simulink model "dds_cwg"  (R2016b)
settings: Solver=VariableStepAuto  StartTime=0.0  StopTime=2048*10  RelTol=1e-3
undefined symbols (not defined in the file or in its folder): fft_stages, n_taps
undefined symbols (not defined in the file): Coeffs, pfb_coeff_gen_calc
libraries: xbsIndex_r4 x6830, casper_library_misc x16, casper_library_delays x2
(part 15 of 67)

== system dds_cwg/DDC/dec_fir_async ==
  sync_in : Inport
  dv_in : Inport  Port=2
  real1 : Inport  Port=3
  imag1 : Inport  Port=4
  real2 : Inport  Port=5
  imag2 : Inport  Port=6
  real3 : Inport  Port=7
  imag3 : Inport  Port=8
  real4 : Inport  Port=9
  imag4 : Inport  Port=10
  real5 : Inport  Port=11
  imag5 : Inport  Port=12
  real6 : Inport  Port=13
  imag6 : Inport  Port=14
  real7 : Inport  Port=15
  imag7 : Inport  Port=16
  real8 : Inport  Port=17
  imag8 : Inport  Port=18
  convert1 : xbsIndex_r4/Convert  gui_display_data_type=Fixed-point  arith_type="Signed  (2's comp)"  n_bits=35  bin_pt=26  float_type=Single  exp_bits=8  fraction_bits=24  quantization="Round  (unbiased: +/- Inf)"  overflow=Wrap  en=off  latency=7  pipeline=off  dbl_ovrd=off  block_type=convert
  convert2 : xbsIndex_r4/Convert  gui_display_data_type=Fixed-point  arith_type="Signed  (2's comp)"  n_bits=35  bin_pt=26  float_type=Single  exp_bits=8  fraction_bits=24  quantization="Round  (unbiased: +/- Inf)"  overflow=Wrap  en=off  latency=7  pipeline=off  dbl_ovrd=off  block_type=convert
  dv_delay : xbsIndex_r4/Delay  rst=off  infoeditControl=Selection of Reset will increase slice count due to use of real FFs and instead of SRLs  en=off  latency=70  reg_retiming=off  dbl_ovrd=off  block_type=delay
      settings: infoedit=Hardware notes: A delay line is a chain, each link of which is an SRL16 or SRL32 followed by a flip-flop.
  fir_col_async1 : Subsystem  AncestorBlock=casper_library_downconverter/fir_col_async  mask(fir_col_async){n_inputs=8, coeff=[-0.0012628 -0.00099956 -0.00074444 -0.00051594 -0.00032729 -0.00018718 -0.00010242  0.00015765], add_latency=7, mult_latency=7, coeff_bit_width=18, coeff_bin_pt=17, first_stage_hdl=on, adder_imp=DSP48, async=on, bus_input=off, input_width=0, input_bp=0, input_type=Signed, dbl=off}
      mask prompts: n_inputs "Inputs"; coeff "Coefficients"; add_latency "Add latency"; mult_latency "Mult Latency"; coeff_bit_width "Coefficient bit width"; coeff_bin_pt "Coefficient binary point"; first_stage_hdl "Implement first stage of adder trees on output as behavioural HDL"; adder_imp "Adder implementation"; async "Asynchronous ops"; bus_input "Bus input"; input_width "Input bitwidth"; input_bp "Input binary point"; input_type "Input datatype"; dbl "Double col"
      mask init:
      | fir_col_async_init(gcb);
      mask Help: eval('xlWeb(''http://casper.berkeley.edu/wiki/Fir_col'')')
      mask TypeOptions adder_imp: Behavioral | Fabric | DSP48
      mask Callback bus_input:
      | onoff = get_param(gcb, 'bus_input');
      | set_param_state(gcb, 'input_width', onoff)
      | set_param_state(gcb, 'input_bp', onoff)
      | set_param_state(gcb, 'input_type', onoff)
      mask TypeOptions input_type: Signed | Unsigned
  fir_col_async10 : Subsystem  AncestorBlock=casper_library_downconverter/fir_col_async  mask(fir_col_async){n_inputs=8, coeff=[0.070166    0.055743    0.040656     0.02581    0.012049  9.3633e-05  -0.0095102   -0.016422], add_latency=7, mult_latency=7, coeff_bit_width=18, coeff_bin_pt=17, first_stage_hdl=on, adder_imp=DSP48, async=on, bus_input=off, input_width=0, input_bp=0, input_type=Signed, dbl=off}
      mask prompts: n_inputs "Inputs"; coeff "Coefficients"; add_latency "Add latency"; mult_latency "Mult Latency"; coeff_bit_width "Coefficient bit width"; coeff_bin_pt "Coefficient binary point"; first_stage_hdl "Implement first stage of adder trees on output as behavioural HDL"; adder_imp "Adder implementation"; async "Asynchronous ops"; bus_input "Bus input"; input_width "Input bitwidth"; input_bp "Input binary point"; input_type "Input datatype"; dbl "Double col"
      mask init:
      | fir_col_async_init(gcb);
      mask Help: eval('xlWeb(''http://casper.berkeley.edu/wiki/Fir_col'')')
      mask TypeOptions adder_imp: Behavioral | Fabric | DSP48
      mask Callback bus_input:
      | onoff = get_param(gcb, 'bus_input');
      | set_param_state(gcb, 'input_width', onoff)
      | set_param_state(gcb, 'input_bp', onoff)
      | set_param_state(gcb, 'input_type', onoff)
      mask TypeOptions input_type: Signed | Unsigned
  fir_col_async11 : Subsystem  AncestorBlock=casper_library_downconverter/fir_col_async  mask(fir_col_async){n_inputs=8, coeff=[0.083023    0.093488     0.10088      0.1047      0.1047     0.10088    0.093488    0.083023], add_latency=7, mult_latency=7, coeff_bit_width=18, coeff_bin_pt=17, first_stage_hdl=on, adder_imp=DSP48, async=on, bus_input=off, input_width=0, input_bp=0, input_type=Signed, dbl=off}
      mask prompts: n_inputs "Inputs"; coeff "Coefficients"; add_latency "Add latency"; mult_latency "Mult Latency"; coeff_bit_width "Coefficient bit width"; coeff_bin_pt "Coefficient binary point"; first_stage_hdl "Implement first stage of adder trees on output as behavioural HDL"; adder_imp "Adder implementation"; async "Asynchronous ops"; bus_input "Bus input"; input_width "Input bitwidth"; input_bp "Input binary point"; input_type "Input datatype"; dbl "Double col"
      mask init:
      | fir_col_async_init(gcb);
      mask Help: eval('xlWeb(''http://casper.berkeley.edu/wiki/Fir_col'')')
      mask TypeOptions adder_imp: Behavioral | Fabric | DSP48
      mask Callback bus_input:
      | onoff = get_param(gcb, 'bus_input');
      | set_param_state(gcb, 'input_width', onoff)
      | set_param_state(gcb, 'input_bp', onoff)
      | set_param_state(gcb, 'input_type', onoff)
      mask TypeOptions input_type: Signed | Unsigned
  fir_col_async12 : Subsystem  AncestorBlock=casper_library_downconverter/fir_col_async  mask(fir_col_async){n_inputs=8, coeff=[-0.016422  -0.0095102  9.3633e-05    0.012049     0.02581    0.040656    0.055743    0.070166], add_latency=7, mult_latency=7, coeff_bit_width=18, coeff_bin_pt=17, first_stage_hdl=on, adder_imp=DSP48, async=on, bus_input=off, input_width=0, input_bp=0, input_type=Signed, dbl=off}
      mask prompts: n_inputs "Inputs"; coeff "Coefficients"; add_latency "Add latency"; mult_latency "Mult Latency"; coeff_bit_width "Coefficient bit width"; coeff_bin_pt "Coefficient binary point"; first_stage_hdl "Implement first stage of adder trees on output as behavioural HDL"; adder_imp "Adder implementation"; async "Asynchronous ops"; bus_input "Bus input"; input_width "Input bitwidth"; input_bp "Input binary point"; input_type "Input datatype"; dbl "Double col"
      mask init:
      | fir_col_async_init(gcb);
      mask Help: eval('xlWeb(''http://casper.berkeley.edu/wiki/Fir_col'')')
      mask TypeOptions adder_imp: Behavioral | Fabric | DSP48
      mask Callback bus_input:
      | onoff = get_param(gcb, 'bus_input');
      | set_param_state(gcb, 'input_width', onoff)
      | set_param_state(gcb, 'input_bp', onoff)
      | set_param_state(gcb, 'input_type', onoff)
      mask TypeOptions input_type: Signed | Unsigned
  fir_col_async13 : Subsystem  AncestorBlock=casper_library_downconverter/fir_col_async  mask(fir_col_async){n_inputs=8, coeff=[0.0023352  -0.0027452  -0.0081837   -0.013424   -0.017857    -0.02087   -0.021908   -0.020523], add_latency=7, mult_latency=7, coeff_bit_width=18, coeff_bin_pt=17, first_stage_hdl=on, adder_imp=DSP48, async=on, bus_input=off, input_width=0, input_bp=0, input_type=Signed, dbl=off}
      mask prompts: n_inputs "Inputs"; coeff "Coefficients"; add_latency "Add latency"; mult_latency "Mult Latency"; coeff_bit_width "Coefficient bit width"; coeff_bin_pt "Coefficient binary point"; first_stage_hdl "Implement first stage of adder trees on output as behavioural HDL"; adder_imp "Adder implementation"; async "Asynchronous ops"; bus_input "Bus input"; input_width "Input bitwidth"; input_bp "Input binary point"; input_type "Input datatype"; dbl "Double col"
      mask init:
      | fir_col_async_init(gcb);
      mask Help: eval('xlWeb(''http://casper.berkeley.edu/wiki/Fir_col'')')
      mask TypeOptions adder_imp: Behavioral | Fabric | DSP48
      mask Callback bus_input:
      | onoff = get_param(gcb, 'bus_input');
      | set_param_state(gcb, 'input_width', onoff)
      | set_param_state(gcb, 'input_bp', onoff)
      | set_param_state(gcb, 'input_type', onoff)
      mask TypeOptions input_type: Signed | Unsigned
  fir_col_async14 : Subsystem  AncestorBlock=casper_library_downconverter/fir_col_async  mask(fir_col_async){n_inputs=8, coeff=[0.0033255   0.0064163   0.0090972    0.011022     0.01189    0.011487     0.00971   0.0065975], add_latency=7, mult_latency=7, coeff_bit_width=18, coeff_bin_pt=17, first_stage_hdl=on, adder_imp=DSP48, async=on, bus_input=off, input_width=0, input_bp=0, input_type=Signed, dbl=off}
      mask prompts: n_inputs "Inputs"; coeff "Coefficients"; add_latency "Add latency"; mult_latency "Mult Latency"; coeff_bit_width "Coefficient bit width"; coeff_bin_pt "Coefficient binary point"; first_stage_hdl "Implement first stage of adder trees on output as behavioural HDL"; adder_imp "Adder implementation"; async "Asynchronous ops"; bus_input "Bus input"; input_width "Input bitwidth"; input_bp "Input binary point"; input_type "Input datatype"; dbl "Double col"
      mask init:
      | fir_col_async_init(gcb);
      mask Help: eval('xlWeb(''http://casper.berkeley.edu/wiki/Fir_col'')')
      mask TypeOptions adder_imp: Behavioral | Fabric | DSP48
      mask Callback bus_input:
      | onoff = get_param(gcb, 'bus_input');
      | set_param_state(gcb, 'input_width', onoff)
      | set_param_state(gcb, 'input_bp', onoff)
      | set_param_state(gcb, 'input_type', onoff)
      mask TypeOptions input_type: Signed | Unsigned
  fir_col_async15 : Subsystem  AncestorBlock=casper_library_downconverter/fir_col_async  mask(fir_col_async){n_inputs=8, coeff=[-0.0050789  -0.0065053  -0.0073276  -0.0073948  -0.0066259  -0.0050262  -0.0026942  0.00017956], add_latency=7, mult_latency=7, coeff_bit_width=18, coeff_bin_pt=17, first_stage_hdl=on, adder_imp=DSP48, async=on, bus_input=off, input_width=0, input_bp=0, input_type=Signed, dbl=off}
      mask prompts: n_inputs "Inputs"; coeff "Coefficients"; add_latency "Add latency"; mult_latency "Mult Latency"; coeff_bit_width "Coefficient bit width"; coeff_bin_pt "Coefficient binary point"; first_stage_hdl "Implement first stage of adder trees on output as behavioural HDL"; adder_imp "Adder implementation"; async "Asynchronous ops"; bus_input "Bus input"; input_width "Input bitwidth"; input_bp "Input binary point"; input_type "Input datatype"; dbl "Double col"
      mask init:
      | fir_col_async_init(gcb);
      mask Help: eval('xlWeb(''http://casper.berkeley.edu/wiki/Fir_col'')')
      mask TypeOptions adder_imp: Behavioral | Fabric | DSP48
      mask Callback bus_input:
      | onoff = get_param(gcb, 'bus_input');
      | set_param_state(gcb, 'input_width', onoff)
      | set_param_state(gcb, 'input_bp', onoff)
      | set_param_state(gcb, 'input_type', onoff)
      mask TypeOptions input_type: Signed | Unsigned
  fir_col_async16 : Subsystem  AncestorBlock=casper_library_downconverter/fir_col_async  mask(fir_col_async){n_inputs=8, coeff=[0.0046187    0.004871   0.0045962   0.0037763   0.0024531  0.00072919  -0.0012378  -0.0032483], add_latency=7, mult_latency=7, coeff_bit_width=18, coeff_bin_pt=17, first_stage_hdl=on, adder_imp=DSP48, async=on, bus_input=off, input_width=0, input_bp=0, input_type=Signed, dbl=off}
      mask prompts: n_inputs "Inputs"; coeff "Coefficients"; add_latency "Add latency"; mult_latency "Mult Latency"; coeff_bit_width "Coefficient bit width"; coeff_bin_pt "Coefficient binary point"; first_stage_hdl "Implement first stage of adder trees on output as behavioural HDL"; adder_imp "Adder implementation"; async "Asynchronous ops"; bus_input "Bus input"; input_width "Input bitwidth"; input_bp "Input binary point"; input_type "Input datatype"; dbl "Double col"
      mask init:
      | fir_col_async_init(gcb);
      mask Help: eval('xlWeb(''http://casper.berkeley.edu/wiki/Fir_col'')')
      mask TypeOptions adder_imp: Behavioral | Fabric | DSP48
      mask Callback bus_input:
      | onoff = get_param(gcb, 'bus_input');
      | set_param_state(gcb, 'input_width', onoff)
      | set_param_state(gcb, 'input_bp', onoff)
      | set_param_state(gcb, 'input_type', onoff)
      mask TypeOptions input_type: Signed | Unsigned
  fir_col_async17 : Subsystem  AncestorBlock=casper_library_downconverter/fir_col_async  mask(fir_col_async){n_inputs=8, coeff=[-0.0031192  -0.0027219  -0.0019821 -0.00095069  0.00028337   0.0015999   0.0028581   0.0039104], add_latency=7, mult_latency=7, coeff_bit_width=18, coeff_bin_pt=17, first_stage_hdl=on, adder_imp=DSP48, async=on, bus_input=off, input_width=0, input_bp=0, input_type=Signed, dbl=off}
      mask prompts: n_inputs "Inputs"; coeff "Coefficients"; add_latency "Add latency"; mult_latency "Mult Latency"; coeff_bit_width "Coefficient bit width"; coeff_bin_pt "Coefficient binary point"; first_stage_hdl "Implement first stage of adder trees on output as behavioural HDL"; adder_imp "Adder implementation"; async "Asynchronous ops"; bus_input "Bus input"; input_width "Input bitwidth"; input_bp "Input binary point"; input_type "Input datatype"; dbl "Double col"
      mask init:
      | fir_col_async_init(gcb);
      mask Help: eval('xlWeb(''http://casper.berkeley.edu/wiki/Fir_col'')')
      mask TypeOptions adder_imp: Behavioral | Fabric | DSP48
      mask Callback bus_input:
      | onoff = get_param(gcb, 'bus_input');
      | set_param_state(gcb, 'input_width', onoff)
      | set_param_state(gcb, 'input_bp', onoff)
      | set_param_state(gcb, 'input_type', onoff)
      mask TypeOptions input_type: Signed | Unsigned
  fir_col_async18 : Subsystem  AncestorBlock=casper_library_downconverter/fir_col_async  mask(fir_col_async){n_inputs=8, coeff=[0.00149  0.00087891  0.00011449 -0.00073276  -0.0015765  -0.0023222  -0.0028776  -0.0031624], add_latency=7, mult_latency=7, coeff_bit_width=18, coeff_bin_pt=17, first_stage_hdl=on, adder_imp=DSP48, async=on, bus_input=off, input_width=0, input_bp=0, input_type=Signed, dbl=off}
      mask prompts: n_inputs "Inputs"; coeff "Coefficients"; add_latency "Add latency"; mult_latency "Mult Latency"; coeff_bit_width "Coefficient bit width"; coeff_bin_pt "Coefficient binary point"; first_stage_hdl "Implement first stage of adder trees on output as behavioural HDL"; adder_imp "Adder implementation"; async "Asynchronous ops"; bus_input "Bus input"; input_width "Input bitwidth"; input_bp "Input binary point"; input_type "Input datatype"; dbl "Double col"
      mask init:
      | fir_col_async_init(gcb);
      mask Help: eval('xlWeb(''http://casper.berkeley.edu/wiki/Fir_col'')')
      mask TypeOptions adder_imp: Behavioral | Fabric | DSP48
      mask Callback bus_input:
      | onoff = get_param(gcb, 'bus_input');
      | set_param_state(gcb, 'input_width', onoff)
      | set_param_state(gcb, 'input_bp', onoff)
      | set_param_state(gcb, 'input_type', onoff)
      mask TypeOptions input_type: Signed | Unsigned
  fir_col_async19 : Subsystem  AncestorBlock=casper_library_downconverter/fir_col_async  mask(fir_col_async){n_inputs=8, coeff=[-0.00030981  0.00027258  0.00085436   0.0013796   0.0017916   0.0020389   0.0020822   0.0018995], add_latency=7, mult_latency=7, coeff_bit_width=18, coeff_bin_pt=17, first_stage_hdl=on, adder_imp=DSP48, async=on, bus_input=off, input_width=0, input_bp=0, input_type=Signed, dbl=off}
      mask prompts: n_inputs "Inputs"; coeff "Coefficients"; add_latency "Add latency"; mult_latency "Mult Latency"; coeff_bit_width "Coefficient bit width"; coeff_bin_pt "Coefficient binary point"; first_stage_hdl "Implement first stage of adder trees on output as behavioural HDL"; adder_imp "Adder implementation"; async "Asynchronous ops"; bus_input "Bus input"; input_width "Input bitwidth"; input_bp "Input binary point"; input_type "Input datatype"; dbl "Double col"
      mask init:
      | fir_col_async_init(gcb);
      mask Help: eval('xlWeb(''http://casper.berkeley.edu/wiki/Fir_col'')')
      mask TypeOptions adder_imp: Behavioral | Fabric | DSP48
      mask Callback bus_input:
      | onoff = get_param(gcb, 'bus_input');
      | set_param_state(gcb, 'input_width', onoff)
      | set_param_state(gcb, 'input_bp', onoff)
      | set_param_state(gcb, 'input_type', onoff)
      mask TypeOptions input_type: Signed | Unsigned
  fir_col_async2 : Subsystem  AncestorBlock=casper_library_downconverter/fir_col_async  mask(fir_col_async){n_inputs=8, coeff=[-0.00084313   -0.001288  -0.0016178  -0.0018198  -0.0018943  -0.0018532  -0.0017168  -0.0015108], add_latency=7, mult_latency=7, coeff_bit_width=18, coeff_bin_pt=17, first_stage_hdl=on, adder_imp=DSP48, async=on, bus_input=off, input_width=0, input_bp=0, input_type=Signed, dbl=off}
      mask prompts: n_inputs "Inputs"; coeff "Coefficients"; add_latency "Add latency"; mult_latency "Mult Latency"; coeff_bit_width "Coefficient bit width"; coeff_bin_pt "Coefficient binary point"; first_stage_hdl "Implement first stage of adder trees on output as behavioural HDL"; adder_imp "Adder implementation"; async "Asynchronous ops"; bus_input "Bus input"; input_width "Input bitwidth"; input_bp "Input binary point"; input_type "Input datatype"; dbl "Double col"
      mask init:
      | fir_col_async_init(gcb);
      mask Help: eval('xlWeb(''http://casper.berkeley.edu/wiki/Fir_col'')')
      mask TypeOptions adder_imp: Behavioral | Fabric | DSP48
      mask Callback bus_input:
      | onoff = get_param(gcb, 'bus_input');
      | set_param_state(gcb, 'input_width', onoff)
      | set_param_state(gcb, 'input_bp', onoff)
      | set_param_state(gcb, 'input_type', onoff)
      mask TypeOptions input_type: Signed | Unsigned
  fir_col_async20 : Subsystem  AncestorBlock=casper_library_downconverter/fir_col_async  mask(fir_col_async){n_inputs=8, coeff=[-0.0015108  -0.0017168  -0.0018532  -0.0018943  -0.0018198  -0.0016178   -0.001288 -0.00084313], add_latency=7, mult_latency=7, coeff_bit_width=18, coeff_bin_pt=17, first_stage_hdl=on, adder_imp=DSP48, async=on, bus_input=off, input_width=0, input_bp=0, input_type=Signed, dbl=off}
      mask prompts: n_inputs "Inputs"; coeff "Coefficients"; add_latency "Add latency"; mult_latency "Mult Latency"; coeff_bit_width "Coefficient bit width"; coeff_bin_pt "Coefficient binary point"; first_stage_hdl "Implement first stage of adder trees on output as behavioural HDL"; adder_imp "Adder implementation"; async "Asynchronous ops"; bus_input "Bus input"; input_width "Input bitwidth"; input_bp "Input binary point"; input_type "Input datatype"; dbl "Double col"
      mask init:
      | fir_col_async_init(gcb);
      mask Help: eval('xlWeb(''http://casper.berkeley.edu/wiki/Fir_col'')')
      mask TypeOptions adder_imp: Behavioral | Fabric | DSP48
      mask Callback bus_input:
      | onoff = get_param(gcb, 'bus_input');
      | set_param_state(gcb, 'input_width', onoff)
      | set_param_state(gcb, 'input_bp', onoff)
      | set_param_state(gcb, 'input_type', onoff)
      mask TypeOptions input_type: Signed | Unsigned
  fir_col_async21 : Subsystem  AncestorBlock=casper_library_downconverter/fir_col_async  mask(fir_col_async){n_inputs=8, coeff=[0.00015765 -0.00010242 -0.00018718 -0.00032729 -0.00051594 -0.00074444 -0.00099956  -0.0012628], add_latency=7, mult_latency=7, coeff_bit_width=18, coeff_bin_pt=17, first_stage_hdl=on, adder_imp=DSP48, async=on, bus_input=off, input_width=0, input_bp=0, input_type=Signed, dbl=off}
      mask prompts: n_inputs "Inputs"; coeff "Coefficients"; add_latency "Add latency"; mult_latency "Mult Latency"; coeff_bit_width "Coefficient bit width"; coeff_bin_pt "Coefficient binary point"; first_stage_hdl "Implement first stage of adder trees on output as behavioural HDL"; adder_imp "Adder implementation"; async "Asynchronous ops"; bus_input "Bus input"; input_width "Input bitwidth"; input_bp "Input binary point"; input_type "Input datatype"; dbl "Double col"
      mask init:
      | fir_col_async_init(gcb);
      mask Help: eval('xlWeb(''http://casper.berkeley.edu/wiki/Fir_col'')')
      mask TypeOptions adder_imp: Behavioral | Fabric | DSP48
      mask Callback bus_input:
      | onoff = get_param(gcb, 'bus_input');
      | set_param_state(gcb, 'input_width', onoff)
      | set_param_state(gcb, 'input_bp', onoff)
      | set_param_state(gcb, 'input_type', onoff)
      mask TypeOptions input_type: Signed | Unsigned
  fir_col_async3 : Subsystem  AncestorBlock=casper_library_downconverter/fir_col_async  mask(fir_col_async){n_inputs=8, coeff=[0.0018995   0.0020822   0.0020389   0.0017916   0.0013796  0.00085436  0.00027258 -0.00030981], add_latency=7, mult_latency=7, coeff_bit_width=18, coeff_bin_pt=17, first_stage_hdl=on, adder_imp=DSP48, async=on, bus_input=off, input_width=0, input_bp=0, input_type=Signed, dbl=off}
      mask prompts: n_inputs "Inputs"; coeff "Coefficients"; add_latency "Add latency"; mult_latency "Mult Latency"; coeff_bit_width "Coefficient bit width"; coeff_bin_pt "Coefficient binary point"; first_stage_hdl "Implement first stage of adder trees on output as behavioural HDL"; adder_imp "Adder implementation"; async "Asynchronous ops"; bus_input "Bus input"; input_width "Input bitwidth"; input_bp "Input binary point"; input_type "Input datatype"; dbl "Double col"
      mask init:
      | fir_col_async_init(gcb);
      mask Help: eval('xlWeb(''http://casper.berkeley.edu/wiki/Fir_col'')')
      mask TypeOptions adder_imp: Behavioral | Fabric | DSP48
      mask Callback bus_input:
      | onoff = get_param(gcb, 'bus_input');
      | set_param_state(gcb, 'input_width', onoff)
      | set_param_state(gcb, 'input_bp', onoff)
      | set_param_state(gcb, 'input_type', onoff)
      mask TypeOptions input_type: Signed | Unsigned
  fir_col_async4 : Subsystem  AncestorBlock=casper_library_downconverter/fir_col_async  mask(fir_col_async){n_inputs=8, coeff=[-0.0031624  -0.0028776  -0.0023222  -0.0015765 -0.00073276  0.00011449  0.00087891     0.00149], add_latency=7, mult_latency=7, coeff_bit_width=18, coeff_bin_pt=17, first_stage_hdl=on, adder_imp=DSP48, async=on, bus_input=off, input_width=0, input_bp=0, input_type=Signed, dbl=off}
      mask prompts: n_inputs "Inputs"; coeff "Coefficients"; add_latency "Add latency"; mult_latency "Mult Latency"; coeff_bit_width "Coefficient bit width"; coeff_bin_pt "Coefficient binary point"; first_stage_hdl "Implement first stage of adder trees on output as behavioural HDL"; adder_imp "Adder implementation"; async "Asynchronous ops"; bus_input "Bus input"; input_width "Input bitwidth"; input_bp "Input binary point"; input_type "Input datatype"; dbl "Double col"
      mask init:
      | fir_col_async_init(gcb);
      mask Help: eval('xlWeb(''http://casper.berkeley.edu/wiki/Fir_col'')')
      mask TypeOptions adder_imp: Behavioral | Fabric | DSP48
      mask Callback bus_input:
      | onoff = get_param(gcb, 'bus_input');
      | set_param_state(gcb, 'input_width', onoff)
      | set_param_state(gcb, 'input_bp', onoff)
      | set_param_state(gcb, 'input_type', onoff)
      mask TypeOptions input_type: Signed | Unsigned
  fir_col_async5 : Subsystem  AncestorBlock=casper_library_downconverter/fir_col_async  mask(fir_col_async){n_inputs=8, coeff=[0.0039104   0.0028581   0.0015999  0.00028337 -0.00095069  -0.0019821  -0.0027219  -0.0031192], add_latency=7, mult_latency=7, coeff_bit_width=18, coeff_bin_pt=17, first_stage_hdl=on, adder_imp=DSP48, async=on, bus_input=off, input_width=0, input_bp=0, input_type=Signed, dbl=off}
      mask prompts: n_inputs "Inputs"; coeff "Coefficients"; add_latency "Add latency"; mult_latency "Mult Latency"; coeff_bit_width "Coefficient bit width"; coeff_bin_pt "Coefficient binary point"; first_stage_hdl "Implement first stage of adder trees on output as behavioural HDL"; adder_imp "Adder implementation"; async "Asynchronous ops"; bus_input "Bus input"; input_width "Input bitwidth"; input_bp "Input binary point"; input_type "Input datatype"; dbl "Double col"
      mask init:
      | fir_col_async_init(gcb);
      mask Help: eval('xlWeb(''http://casper.berkeley.edu/wiki/Fir_col'')')
      mask TypeOptions adder_imp: Behavioral | Fabric | DSP48
      mask Callback bus_input:
      | onoff = get_param(gcb, 'bus_input');
      | set_param_state(gcb, 'input_width', onoff)
      | set_param_state(gcb, 'input_bp', onoff)
      | set_param_state(gcb, 'input_type', onoff)
      mask TypeOptions input_type: Signed | Unsigned
  fir_col_async6 : Subsystem  AncestorBlock=casper_library_downconverter/fir_col_async  mask(fir_col_async){n_inputs=8, coeff=[-0.0032483  -0.0012378  0.00072919   0.0024531   0.0037763   0.0045962    0.004871   0.0046187], add_latency=7, mult_latency=7, coeff_bit_width=18, coeff_bin_pt=17, first_stage_hdl=on, adder_imp=DSP48, async=on, bus_input=off, input_width=0, input_bp=0, input_type=Signed, dbl=off}
      mask prompts: n_inputs "Inputs"; coeff "Coefficients"; add_latency "Add latency"; mult_latency "Mult Latency"; coeff_bit_width "Coefficient bit width"; coeff_bin_pt "Coefficient binary point"; first_stage_hdl "Implement first stage of adder trees on output as behavioural HDL"; adder_imp "Adder implementation"; async "Asynchronous ops"; bus_input "Bus input"; input_width "Input bitwidth"; input_bp "Input binary point"; input_type "Input datatype"; dbl "Double col"
      mask init:
      | fir_col_async_init(gcb);
      mask Help: eval('xlWeb(''http://casper.berkeley.edu/wiki/Fir_col'')')
      mask TypeOptions adder_imp: Behavioral | Fabric | DSP48
      mask Callback bus_input:
      | onoff = get_param(gcb, 'bus_input');
      | set_param_state(gcb, 'input_width', onoff)
      | set_param_state(gcb, 'input_bp', onoff)
      | set_param_state(gcb, 'input_type', onoff)
      mask TypeOptions input_type: Signed | Unsigned
  fir_col_async7 : Subsystem  AncestorBlock=casper_library_downconverter/fir_col_async  mask(fir_col_async){n_inputs=8, coeff=[0.00017956  -0.0026942  -0.0050262  -0.0066259  -0.0073948  -0.0073276  -0.0065053  -0.0050789], add_latency=7, mult_latency=7, coeff_bit_width=18, coeff_bin_pt=17, first_stage_hdl=on, adder_imp=DSP48, async=on, bus_input=off, input_width=0, input_bp=0, input_type=Signed, dbl=off}
      mask prompts: n_inputs "Inputs"; coeff "Coefficients"; add_latency "Add latency"; mult_latency "Mult Latency"; coeff_bit_width "Coefficient bit width"; coeff_bin_pt "Coefficient binary point"; first_stage_hdl "Implement first stage of adder trees on output as behavioural HDL"; adder_imp "Adder implementation"; async "Asynchronous ops"; bus_input "Bus input"; input_width "Input bitwidth"; input_bp "Input binary point"; input_type "Input datatype"; dbl "Double col"
      mask init:
      | fir_col_async_init(gcb);
      mask Help: eval('xlWeb(''http://casper.berkeley.edu/wiki/Fir_col'')')
      mask TypeOptions adder_imp: Behavioral | Fabric | DSP48
      mask Callback bus_input:
      | onoff = get_param(gcb, 'bus_input');
      | set_param_state(gcb, 'input_width', onoff)
      | set_param_state(gcb, 'input_bp', onoff)
      | set_param_state(gcb, 'input_type', onoff)
      mask TypeOptions input_type: Signed | Unsigned
  fir_col_async8 : Subsystem  AncestorBlock=casper_library_downconverter/fir_col_async  mask(fir_col_async){n_inputs=8, coeff=[0.0065975     0.00971    0.011487     0.01189    0.011022   0.0090972   0.0064163   0.0033255], add_latency=7, mult_latency=7, coeff_bit_width=18, coeff_bin_pt=17, first_stage_hdl=on, adder_imp=DSP48, async=on, bus_input=off, input_width=0, input_bp=0, input_type=Signed, dbl=off}
      mask prompts: n_inputs "Inputs"; coeff "Coefficients"; add_latency "Add latency"; mult_latency "Mult Latency"; coeff_bit_width "Coefficient bit width"; coeff_bin_pt "Coefficient binary point"; first_stage_hdl "Implement first stage of adder trees on output as behavioural HDL"; adder_imp "Adder implementation"; async "Asynchronous ops"; bus_input "Bus input"; input_width "Input bitwidth"; input_bp "Input binary point"; input_type "Input datatype"; dbl "Double col"
      mask init:
      | fir_col_async_init(gcb);
      mask Help: eval('xlWeb(''http://casper.berkeley.edu/wiki/Fir_col'')')
      mask TypeOptions adder_imp: Behavioral | Fabric | DSP48
      mask Callback bus_input:
      | onoff = get_param(gcb, 'bus_input');
      | set_param_state(gcb, 'input_width', onoff)
      | set_param_state(gcb, 'input_bp', onoff)
      | set_param_state(gcb, 'input_type', onoff)
      mask TypeOptions input_type: Signed | Unsigned
  fir_col_async9 : Subsystem  AncestorBlock=casper_library_downconverter/fir_col_async  mask(fir_col_async){n_inputs=8, coeff=[-0.020523   -0.021908    -0.02087   -0.017857   -0.013424  -0.0081837  -0.0027452   0.0023352], add_latency=7, mult_latency=7, coeff_bit_width=18, coeff_bin_pt=17, first_stage_hdl=on, adder_imp=DSP48, async=on, bus_input=off, input_width=0, input_bp=0, input_type=Signed, dbl=off}
      mask prompts: n_inputs "Inputs"; coeff "Coefficients"; add_latency "Add latency"; mult_latency "Mult Latency"; coeff_bit_width "Coefficient bit width"; coeff_bin_pt "Coefficient binary point"; first_stage_hdl "Implement first stage of adder trees on output as behavioural HDL"; adder_imp "Adder implementation"; async "Asynchronous ops"; bus_input "Bus input"; input_width "Input bitwidth"; input_bp "Input binary point"; input_type "Input datatype"; dbl "Double col"
      mask init:
      | fir_col_async_init(gcb);
      mask Help: eval('xlWeb(''http://casper.berkeley.edu/wiki/Fir_col'')')
      mask TypeOptions adder_imp: Behavioral | Fabric | DSP48
      mask Callback bus_input:
      | onoff = get_param(gcb, 'bus_input');
      | set_param_state(gcb, 'input_width', onoff)
      | set_param_state(gcb, 'input_bp', onoff)
      | set_param_state(gcb, 'input_type', onoff)
      mask TypeOptions input_type: Signed | Unsigned
  imag_sum : Subsystem  AncestorBlock=casper_library_misc/adder_tree  mask(adder_tree){n_inputs=21, latency=7, adder_imp=DSP48, first_stage_hdl=off, floating_point=off, float_type=single, frac_width=0, exp_width=0}
      mask prompts: n_inputs "Number of Inputs"; latency "Add Latency"; adder_imp "Adder implementation"; first_stage_hdl "Use behavioural HDL for first stage of adders"; floating_point "floating point"; float_type "float type"; frac_width "fraction length"; exp_width "exponent length"
      mask help:
      | Sums all inputs using a tree of adds and delays.
      |
      | Number of inputs: The number of inputs to the block to be summed
      | Add latency: The number of clock cycles to perform one addition (affects timing)..
      | Adder implementation: choice of fabric or DSP48E core, or behavioral HDL
      | Use behavioural HDL for first stage of adders: Causes the first stage of adders to be absorbed into DSP blocks if multipliers precede them (Virtex 5). Overrides Adder implementation
      mask init:
      | adder_tree_init(gcb, ...
      |     'n_inputs', n_inputs, ...
      |     'latency', latency, ...
      |     'adder_imp', adder_imp, ...
      |     'floating_point', floating_point, ...
      |     'float_type', float_type, ...
      |     'exp_width', exp_width, ...
      |     'frac_width', frac_width, ...     
      |     'first_stage_hdl', first_stage_hdl);
      settings: AttributesFormatString=latency 35
      mask Help: eval('xlWeb(''http://casper.berkeley.edu/wiki/Adder_tree'')')
      mask TypeOptions adder_imp: Behavioral | Fabric | DSP48
      mask Callback floating_point:
      | onoff = get_param(gcb, 'floating_point');
      | if strcmp(onoff,'on')
      |     enable_fixpt = 'off'
      |     set_param_state(gcb, 'float_type', 'on')
      | 
      |     f_type = get_param(gcb, 'float_type')
      |     if strcmp(f_type,'custom')
      |         set_param_state(gcb, 'exp_width', 'on')
      |         set_param_state(gcb, 'frac_width', 'on')
      |     else
      |         set_param_state(gcb, 'exp_width', 'off')
      |         set_param_state(gcb, 'frac_width', 'off')
      |     end
      | 
      | 
      | else
      |     enable_fixpt = 'on'
      |     set_param_state(gcb, 'float_type', 'off')
      |     set_param_state(gcb, 'exp_width', 'off')
      |     set_param_state(gcb, 'frac_width', 'off')
      | end
      mask TypeOptions float_type: single | custom
      mask Callback float_type:
      | f_type = get_param(gcb, 'float_type')
      | if strcmp(f_type,'custom')
      |     set_param_state(gcb, 'exp_width', 'on')
      |     set_param_state(gcb, 'frac_width', 'on')
      | else
      |     set_param_state(gcb, 'exp_width', 'off')
      |     set_param_state(gcb, 'frac_width', 'off')
      | end
  real_sum : Subsystem  AncestorBlock=casper_library_misc/adder_tree  mask(adder_tree){n_inputs=21, latency=7, adder_imp=DSP48, first_stage_hdl=off, floating_point=off, float_type=single, frac_width=0, exp_width=0}
      mask prompts: n_inputs "Number of Inputs"; latency "Add Latency"; adder_imp "Adder implementation"; first_stage_hdl "Use behavioural HDL for first stage of adders"; floating_point "floating point"; float_type "float type"; frac_width "fraction length"; exp_width "exponent length"
      mask help:
      | Sums all inputs using a tree of adds and delays.
      |
      | Number of inputs: The number of inputs to the block to be summed
      | Add latency: The number of clock cycles to perform one addition (affects timing)..
      | Adder implementation: choice of fabric or DSP48E core, or behavioral HDL
      | Use behavioural HDL for first stage of adders: Causes the first stage of adders to be absorbed into DSP blocks if multipliers precede them (Virtex 5). Overrides Adder implementation
      mask init: same as dds_cwg/DDC/dec_fir_async/imag_sum
      settings: AttributesFormatString=latency 35
      mask Help: eval('xlWeb(''http://casper.berkeley.edu/wiki/Adder_tree'')')
      mask TypeOptions adder_imp: Behavioral | Fabric | DSP48
      mask Callback floating_point:
      | onoff = get_param(gcb, 'floating_point');
      | if strcmp(onoff,'on')
      |     enable_fixpt = 'off'
      |     set_param_state(gcb, 'float_type', 'on')
      | 
      |     f_type = get_param(gcb, 'float_type')
      |     if strcmp(f_type,'custom')
      |         set_param_state(gcb, 'exp_width', 'on')
      |         set_param_state(gcb, 'frac_width', 'on')
      |     else
      |         set_param_state(gcb, 'exp_width', 'off')
      |         set_param_state(gcb, 'frac_width', 'off')
      |     end
      | 
      | 
      | else
      |     enable_fixpt = 'on'
      |     set_param_state(gcb, 'float_type', 'off')
      |     set_param_state(gcb, 'exp_width', 'off')
      |     set_param_state(gcb, 'frac_width', 'off')
      | end
      mask TypeOptions float_type: single | custom
      mask Callback float_type:
      | f_type = get_param(gcb, 'float_type')
      | if strcmp(f_type,'custom')
      |     set_param_state(gcb, 'exp_width', 'on')
      |     set_param_state(gcb, 'frac_width', 'on')
      | else
      |     set_param_state(gcb, 'exp_width', 'off')
      |     set_param_state(gcb, 'frac_width', 'off')
      | end
  ri_to_c : casper_library_misc/ri_to_c
  shift1 : xbsIndex_r4/Shift  shift_dir=Left  shift_bits=1  en=off  latency=1  precision=Full  arith_type="Signed  (2's comp)"  n_bits=16  bin_pt=14  quantization=Truncate  overflow=Wrap  dbl_ovrd=off  block_type=shift
  shift2 : xbsIndex_r4/Shift  shift_dir=Left  shift_bits=1  en=off  latency=1  precision=Full  arith_type="Signed  (2's comp)"  n_bits=16  bin_pt=14  quantization=Truncate  overflow=Wrap  dbl_ovrd=off  block_type=shift
  sync_delay : xbsIndex_r4/Delay  rst=off  infoeditControl=Selection of Reset will increase slice count due to use of real FFs and instead of SRLs  en=off  latency=35  reg_retiming=off  dbl_ovrd=off  block_type=delay
      settings: infoedit=Hardware notes: A delay line is a chain, each link of which is an SRL16 or SRL32 followed by a flip-flop.
  sync_out : Outport
  dout : Outport  Port=2
  dv_out : Outport  Port=3
  wires:
  sync_in/1 -> sync_delay/1
  dv_in/1 -> dv_delay/1, fir_col_async1/17(dv), fir_col_async2/17(dv), fir_col_async3/17(dv), fir_col_async4/17(dv), fir_col_async5/17(dv), fir_col_async6/17(dv), fir_col_async7/17(dv), fir_col_async8/17(dv), fir_col_async9/17(dv), fir_col_async10/17(dv), fir_col_async11/17(dv), fir_col_async12/17(dv), fir_col_async13/17(dv), fir_col_async14/17(dv), fir_col_async15/17(dv), fir_col_async16/17(dv), fir_col_async17/17(dv), fir_col_async18/17(dv), fir_col_async19/17(dv), fir_col_async20/17(dv), fir_col_async21/17(dv)
  dv_delay/1 -> dv_out/1
  real1/1 -> fir_col_async1/1(real1)
  imag1/1 -> fir_col_async1/2(imag1)
  real2/1 -> fir_col_async1/3(real2)
  imag2/1 -> fir_col_async1/4(imag2)
  real3/1 -> fir_col_async1/5(real3)
  imag3/1 -> fir_col_async1/6(imag3)
  real4/1 -> fir_col_async1/7(real4)
  imag4/1 -> fir_col_async1/8(imag4)
  real5/1 -> fir_col_async1/9(real5)
  imag5/1 -> fir_col_async1/10(imag5)
  real6/1 -> fir_col_async1/11(real6)
  imag6/1 -> fir_col_async1/12(imag6)
  real7/1 -> fir_col_async1/13(real7)
  imag7/1 -> fir_col_async1/14(imag7)
  real8/1 -> fir_col_async1/15(real8)
  imag8/1 -> fir_col_async1/16(imag8)
  fir_col_async1/17(real_sum) -> real_sum/2(din1)
  fir_col_async1/18(imag_sum) -> imag_sum/2(din1)
  fir_col_async1/1(real_out1) -> fir_col_async2/1(real1)
  fir_col_async1/2(imag_out1) -> fir_col_async2/2(imag1)
  fir_col_async1/3(real_out2) -> fir_col_async2/3(real2)
  fir_col_async1/4(imag_out2) -> fir_col_async2/4(imag2)
  fir_col_async1/5(real_out3) -> fir_col_async2/5(real3)
  fir_col_async1/6(imag_out3) -> fir_col_async2/6(imag3)
  fir_col_async1/7(real_out4) -> fir_col_async2/7(real4)
  fir_col_async1/8(imag_out4) -> fir_col_async2/8(imag4)
  fir_col_async1/9(real_out5) -> fir_col_async2/9(real5)
  fir_col_async1/10(imag_out5) -> fir_col_async2/10(imag5)
  fir_col_async1/11(real_out6) -> fir_col_async2/11(real6)
  fir_col_async1/12(imag_out6) -> fir_col_async2/12(imag6)
  fir_col_async1/13(real_out7) -> fir_col_async2/13(real7)
  fir_col_async1/14(imag_out7) -> fir_col_async2/14(imag7)
  fir_col_async1/15(real_out8) -> fir_col_async2/15(real8)
  fir_col_async1/16(imag_out8) -> fir_col_async2/16(imag8)
  fir_col_async2/17(real_sum) -> real_sum/3(din2)
  fir_col_async2/18(imag_sum) -> imag_sum/3(din2)
  fir_col_async2/1(real_out1) -> fir_col_async3/1(real1)
  fir_col_async2/2(imag_out1) -> fir_col_async3/2(imag1)
  fir_col_async2/3(real_out2) -> fir_col_async3/3(real2)
  fir_col_async2/4(imag_out2) -> fir_col_async3/4(imag2)
  fir_col_async2/5(real_out3) -> fir_col_async3/5(real3)
  fir_col_async2/6(imag_out3) -> fir_col_async3/6(imag3)
  fir_col_async2/7(real_out4) -> fir_col_async3/7(real4)
  fir_col_async2/8(imag_out4) -> fir_col_async3/8(imag4)
  fir_col_async2/9(real_out5) -> fir_col_async3/9(real5)
  fir_col_async2/10(imag_out5) -> fir_col_async3/10(imag5)
  fir_col_async2/11(real_out6) -> fir_col_async3/11(real6)
  fir_col_async2/12(imag_out6) -> fir_col_async3/12(imag6)
  fir_col_async2/13(real_out7) -> fir_col_async3/13(real7)
  fir_col_async2/14(imag_out7) -> fir_col_async3/14(imag7)
  fir_col_async2/15(real_out8) -> fir_col_async3/15(real8)
  fir_col_async2/16(imag_out8) -> fir_col_async3/16(imag8)
  fir_col_async3/17(real_sum) -> real_sum/4(din3)
  fir_col_async3/18(imag_sum) -> imag_sum/4(din3)
  fir_col_async3/1(real_out1) -> fir_col_async4/1(real1)
  fir_col_async3/2(imag_out1) -> fir_col_async4/2(imag1)
  fir_col_async3/3(real_out2) -> fir_col_async4/3(real2)
  fir_col_async3/4(imag_out2) -> fir_col_async4/4(imag2)
  fir_col_async3/5(real_out3) -> fir_col_async4/5(real3)
  fir_col_async3/6(imag_out3) -> fir_col_async4/6(imag3)
  fir_col_async3/7(real_out4) -> fir_col_async4/7(real4)
  fir_col_async3/8(imag_out4) -> fir_col_async4/8(imag4)
  fir_col_async3/9(real_out5) -> fir_col_async4/9(real5)
  fir_col_async3/10(imag_out5) -> fir_col_async4/10(imag5)
  fir_col_async3/11(real_out6) -> fir_col_async4/11(real6)
  fir_col_async3/12(imag_out6) -> fir_col_async4/12(imag6)
  fir_col_async3/13(real_out7) -> fir_col_async4/13(real7)
  fir_col_async3/14(imag_out7) -> fir_col_async4/14(imag7)
  fir_col_async3/15(real_out8) -> fir_col_async4/15(real8)
  fir_col_async3/16(imag_out8) -> fir_col_async4/16(imag8)
  fir_col_async4/17(real_sum) -> real_sum/5(din4)
  fir_col_async4/18(imag_sum) -> imag_sum/5(din4)
  fir_col_async4/1(real_out1) -> fir_col_async5/1(real1)
  fir_col_async4/2(imag_out1) -> fir_col_async5/2(imag1)
  fir_col_async4/3(real_out2) -> fir_col_async5/3(real2)
  fir_col_async4/4(imag_out2) -> fir_col_async5/4(imag2)
  fir_col_async4/5(real_out3) -> fir_col_async5/5(real3)
  fir_col_async4/6(imag_out3) -> fir_col_async5/6(imag3)
  fir_col_async4/7(real_out4) -> fir_col_async5/7(real4)
  fir_col_async4/8(imag_out4) -> fir_col_async5/8(imag4)
  fir_col_async4/9(real_out5) -> fir_col_async5/9(real5)
  fir_col_async4/10(imag_out5) -> fir_col_async5/10(imag5)
  fir_col_async4/11(real_out6) -> fir_col_async5/11(real6)
  fir_col_async4/12(imag_out6) -> fir_col_async5/12(imag6)
  fir_col_async4/13(real_out7) -> fir_col_async5/13(real7)
  fir_col_async4/14(imag_out7) -> fir_col_async5/14(imag7)
  fir_col_async4/15(real_out8) -> fir_col_async5/15(real8)
  fir_col_async4/16(imag_out8) -> fir_col_async5/16(imag8)
  fir_col_async5/17(real_sum) -> real_sum/6(din5)
  fir_col_async5/18(imag_sum) -> imag_sum/6(din5)
  fir_col_async5/1(real_out1) -> fir_col_async6/1(real1)
  fir_col_async5/2(imag_out1) -> fir_col_async6/2(imag1)
  fir_col_async5/3(real_out2) -> fir_col_async6/3(real2)
  fir_col_async5/4(imag_out2) -> fir_col_async6/4(imag2)
  fir_col_async5/5(real_out3) -> fir_col_async6/5(real3)
  fir_col_async5/6(imag_out3) -> fir_col_async6/6(imag3)
  fir_col_async5/7(real_out4) -> fir_col_async6/7(real4)
  fir_col_async5/8(imag_out4) -> fir_col_async6/8(imag4)
  fir_col_async5/9(real_out5) -> fir_col_async6/9(real5)
  fir_col_async5/10(imag_out5) -> fir_col_async6/10(imag5)
  fir_col_async5/11(real_out6) -> fir_col_async6/11(real6)
  fir_col_async5/12(imag_out6) -> fir_col_async6/12(imag6)
  fir_col_async5/13(real_out7) -> fir_col_async6/13(real7)
  fir_col_async5/14(imag_out7) -> fir_col_async6/14(imag7)
  fir_col_async5/15(real_out8) -> fir_col_async6/15(real8)
  fir_col_async5/16(imag_out8) -> fir_col_async6/16(imag8)
  fir_col_async6/17(real_sum) -> real_sum/7(din6)
  fir_col_async6/18(imag_sum) -> imag_sum/7(din6)
  fir_col_async6/1(real_out1) -> fir_col_async7/1(real1)
  fir_col_async6/2(imag_out1) -> fir_col_async7/2(imag1)
  fir_col_async6/3(real_out2) -> fir_col_async7/3(real2)
  fir_col_async6/4(imag_out2) -> fir_col_async7/4(imag2)
  fir_col_async6/5(real_out3) -> fir_col_async7/5(real3)
  fir_col_async6/6(imag_out3) -> fir_col_async7/6(imag3)
  fir_col_async6/7(real_out4) -> fir_col_async7/7(real4)
  fir_col_async6/8(imag_out4) -> fir_col_async7/8(imag4)
  fir_col_async6/9(real_out5) -> fir_col_async7/9(real5)
  fir_col_async6/10(imag_out5) -> fir_col_async7/10(imag5)
  fir_col_async6/11(real_out6) -> fir_col_async7/11(real6)
  fir_col_async6/12(imag_out6) -> fir_col_async7/12(imag6)
  fir_col_async6/13(real_out7) -> fir_col_async7/13(real7)
  fir_col_async6/14(imag_out7) -> fir_col_async7/14(imag7)
  fir_col_async6/15(real_out8) -> fir_col_async7/15(real8)
  fir_col_async6/16(imag_out8) -> fir_col_async7/16(imag8)
  fir_col_async7/17(real_sum) -> real_sum/8(din7)
  fir_col_async7/18(imag_sum) -> imag_sum/8(din7)
  fir_col_async7/1(real_out1) -> fir_col_async8/1(real1)
  fir_col_async7/2(imag_out1) -> fir_col_async8/2(imag1)
  fir_col_async7/3(real_out2) -> fir_col_async8/3(real2)
  fir_col_async7/4(imag_out2) -> fir_col_async8/4(imag2)
  fir_col_async7/5(real_out3) -> fir_col_async8/5(real3)
  fir_col_async7/6(imag_out3) -> fir_col_async8/6(imag3)
  fir_col_async7/7(real_out4) -> fir_col_async8/7(real4)
  fir_col_async7/8(imag_out4) -> fir_col_async8/8(imag4)
  fir_col_async7/9(real_out5) -> fir_col_async8/9(real5)
  fir_col_async7/10(imag_out5) -> fir_col_async8/10(imag5)
  fir_col_async7/11(real_out6) -> fir_col_async8/11(real6)
  fir_col_async7/12(imag_out6) -> fir_col_async8/12(imag6)
  fir_col_async7/13(real_out7) -> fir_col_async8/13(real7)
  fir_col_async7/14(imag_out7) -> fir_col_async8/14(imag7)
  fir_col_async7/15(real_out8) -> fir_col_async8/15(real8)
  fir_col_async7/16(imag_out8) -> fir_col_async8/16(imag8)
  fir_col_async8/17(real_sum) -> real_sum/9(din8)
  fir_col_async8/18(imag_sum) -> imag_sum/9(din8)
  fir_col_async8/1(real_out1) -> fir_col_async9/1(real1)
  fir_col_async8/2(imag_out1) -> fir_col_async9/2(imag1)
  fir_col_async8/3(real_out2) -> fir_col_async9/3(real2)
  fir_col_async8/4(imag_out2) -> fir_col_async9/4(imag2)
  fir_col_async8/5(real_out3) -> fir_col_async9/5(real3)
  fir_col_async8/6(imag_out3) -> fir_col_async9/6(imag3)
  fir_col_async8/7(real_out4) -> fir_col_async9/7(real4)
  fir_col_async8/8(imag_out4) -> fir_col_async9/8(imag4)
  fir_col_async8/9(real_out5) -> fir_col_async9/9(real5)
  fir_col_async8/10(imag_out5) -> fir_col_async9/10(imag5)
  fir_col_async8/11(real_out6) -> fir_col_async9/11(real6)
  fir_col_async8/12(imag_out6) -> fir_col_async9/12(imag6)
  fir_col_async8/13(real_out7) -> fir_col_async9/13(real7)
  fir_col_async8/14(imag_out7) -> fir_col_async9/14(imag7)
  fir_col_async8/15(real_out8) -> fir_col_async9/15(real8)
  fir_col_async8/16(imag_out8) -> fir_col_async9/16(imag8)
  fir_col_async9/17(real_sum) -> real_sum/10(din9)
  fir_col_async9/18(imag_sum) -> imag_sum/10(din9)
  fir_col_async9/1(real_out1) -> fir_col_async10/1(real1)
  fir_col_async9/2(imag_out1) -> fir_col_async10/2(imag1)
  fir_col_async9/3(real_out2) -> fir_col_async10/3(real2)
  fir_col_async9/4(imag_out2) -> fir_col_async10/4(imag2)
  fir_col_async9/5(real_out3) -> fir_col_async10/5(real3)
  fir_col_async9/6(imag_out3) -> fir_col_async10/6(imag3)
  fir_col_async9/7(real_out4) -> fir_col_async10/7(real4)
  fir_col_async9/8(imag_out4) -> fir_col_async10/8(imag4)
  fir_col_async9/9(real_out5) -> fir_col_async10/9(real5)
  fir_col_async9/10(imag_out5) -> fir_col_async10/10(imag5)
  fir_col_async9/11(real_out6) -> fir_col_async10/11(real6)
  fir_col_async9/12(imag_out6) -> fir_col_async10/12(imag6)
  fir_col_async9/13(real_out7) -> fir_col_async10/13(real7)
  fir_col_async9/14(imag_out7) -> fir_col_async10/14(imag7)
  fir_col_async9/15(real_out8) -> fir_col_async10/15(real8)
  fir_col_async9/16(imag_out8) -> fir_col_async10/16(imag8)
  fir_col_async10/17(real_sum) -> real_sum/11(din10)
  fir_col_async10/18(imag_sum) -> imag_sum/11(din10)
  fir_col_async10/1(real_out1) -> fir_col_async11/1(real1)
  fir_col_async10/2(imag_out1) -> fir_col_async11/2(imag1)
  fir_col_async10/3(real_out2) -> fir_col_async11/3(real2)
  fir_col_async10/4(imag_out2) -> fir_col_async11/4(imag2)
  fir_col_async10/5(real_out3) -> fir_col_async11/5(real3)
  fir_col_async10/6(imag_out3) -> fir_col_async11/6(imag3)
  fir_col_async10/7(real_out4) -> fir_col_async11/7(real4)
  fir_col_async10/8(imag_out4) -> fir_col_async11/8(imag4)
  fir_col_async10/9(real_out5) -> fir_col_async11/9(real5)
  fir_col_async10/10(imag_out5) -> fir_col_async11/10(imag5)
  fir_col_async10/11(real_out6) -> fir_col_async11/11(real6)
  fir_col_async10/12(imag_out6) -> fir_col_async11/12(imag6)
  fir_col_async10/13(real_out7) -> fir_col_async11/13(real7)
  fir_col_async10/14(imag_out7) -> fir_col_async11/14(imag7)
  fir_col_async10/15(real_out8) -> fir_col_async11/15(real8)
  fir_col_async10/16(imag_out8) -> fir_col_async11/16(imag8)
  fir_col_async11/17(real_sum) -> real_sum/12(din11)
  fir_col_async11/18(imag_sum) -> imag_sum/12(din11)
  fir_col_async11/1(real_out1) -> fir_col_async12/1(real1)
  fir_col_async11/2(imag_out1) -> fir_col_async12/2(imag1)
  fir_col_async11/3(real_out2) -> fir_col_async12/3(real2)
  fir_col_async11/4(imag_out2) -> fir_col_async12/4(imag2)
  fir_col_async11/5(real_out3) -> fir_col_async12/5(real3)
  fir_col_async11/6(imag_out3) -> fir_col_async12/6(imag3)
  fir_col_async11/7(real_out4) -> fir_col_async12/7(real4)
  fir_col_async11/8(imag_out4) -> fir_col_async12/8(imag4)
  fir_col_async11/9(real_out5) -> fir_col_async12/9(real5)
  fir_col_async11/10(imag_out5) -> fir_col_async12/10(imag5)
  fir_col_async11/11(real_out6) -> fir_col_async12/11(real6)
  fir_col_async11/12(imag_out6) -> fir_col_async12/12(imag6)
  fir_col_async11/13(real_out7) -> fir_col_async12/13(real7)
  fir_col_async11/14(imag_out7) -> fir_col_async12/14(imag7)
  fir_col_async11/15(real_out8) -> fir_col_async12/15(real8)
  fir_col_async11/16(imag_out8) -> fir_col_async12/16(imag8)
  fir_col_async12/17(real_sum) -> real_sum/13(din12)
  fir_col_async12/18(imag_sum) -> imag_sum/13(din12)
  fir_col_async12/1(real_out1) -> fir_col_async13/1(real1)
  fir_col_async12/2(imag_out1) -> fir_col_async13/2(imag1)
  fir_col_async12/3(real_out2) -> fir_col_async13/3(real2)
  fir_col_async12/4(imag_out2) -> fir_col_async13/4(imag2)
  fir_col_async12/5(real_out3) -> fir_col_async13/5(real3)
  fir_col_async12/6(imag_out3) -> fir_col_async13/6(imag3)
  fir_col_async12/7(real_out4) -> fir_col_async13/7(real4)
  fir_col_async12/8(imag_out4) -> fir_col_async13/8(imag4)
  fir_col_async12/9(real_out5) -> fir_col_async13/9(real5)
  fir_col_async12/10(imag_out5) -> fir_col_async13/10(imag5)
  fir_col_async12/11(real_out6) -> fir_col_async13/11(real6)
  fir_col_async12/12(imag_out6) -> fir_col_async13/12(imag6)
  fir_col_async12/13(real_out7) -> fir_col_async13/13(real7)
  fir_col_async12/14(imag_out7) -> fir_col_async13/14(imag7)
  fir_col_async12/15(real_out8) -> fir_col_async13/15(real8)
  fir_col_async12/16(imag_out8) -> fir_col_async13/16(imag8)
  fir_col_async13/17(real_sum) -> real_sum/14(din13)
  fir_col_async13/18(imag_sum) -> imag_sum/14(din13)
  fir_col_async13/1(real_out1) -> fir_col_async14/1(real1)
  fir_col_async13/2(imag_out1) -> fir_col_async14/2(imag1)
  fir_col_async13/3(real_out2) -> fir_col_async14/3(real2)
  fir_col_async13/4(imag_out2) -> fir_col_async14/4(imag2)
  fir_col_async13/5(real_out3) -> fir_col_async14/5(real3)
  fir_col_async13/6(imag_out3) -> fir_col_async14/6(imag3)
  fir_col_async13/7(real_out4) -> fir_col_async14/7(real4)
  fir_col_async13/8(imag_out4) -> fir_col_async14/8(imag4)
  fir_col_async13/9(real_out5) -> fir_col_async14/9(real5)
  fir_col_async13/10(imag_out5) -> fir_col_async14/10(imag5)
  fir_col_async13/11(real_out6) -> fir_col_async14/11(real6)
  fir_col_async13/12(imag_out6) -> fir_col_async14/12(imag6)
  fir_col_async13/13(real_out7) -> fir_col_async14/13(real7)
  fir_col_async13/14(imag_out7) -> fir_col_async14/14(imag7)
  fir_col_async13/15(real_out8) -> fir_col_async14/15(real8)
  fir_col_async13/16(imag_out8) -> fir_col_async14/16(imag8)
  fir_col_async14/17(real_sum) -> real_sum/15(din14)
  fir_col_async14/18(imag_sum) -> imag_sum/15(din14)
  fir_col_async14/1(real_out1) -> fir_col_async15/1(real1)
  fir_col_async14/2(imag_out1) -> fir_col_async15/2(imag1)
  fir_col_async14/3(real_out2) -> fir_col_async15/3(real2)
  fir_col_async14/4(imag_out2) -> fir_col_async15/4(imag2)
  fir_col_async14/5(real_out3) -> fir_col_async15/5(real3)
  fir_col_async14/6(imag_out3) -> fir_col_async15/6(imag3)
  fir_col_async14/7(real_out4) -> fir_col_async15/7(real4)
  fir_col_async14/8(imag_out4) -> fir_col_async15/8(imag4)
  fir_col_async14/9(real_out5) -> fir_col_async15/9(real5)
  fir_col_async14/10(imag_out5) -> fir_col_async15/10(imag5)
  fir_col_async14/11(real_out6) -> fir_col_async15/11(real6)
  fir_col_async14/12(imag_out6) -> fir_col_async15/12(imag6)
  fir_col_async14/13(real_out7) -> fir_col_async15/13(real7)
  fir_col_async14/14(imag_out7) -> fir_col_async15/14(imag7)
  fir_col_async14/15(real_out8) -> fir_col_async15/15(real8)
  fir_col_async14/16(imag_out8) -> fir_col_async15/16(imag8)
  fir_col_async15/17(real_sum) -> real_sum/16(din15)
  fir_col_async15/18(imag_sum) -> imag_sum/16(din15)
  fir_col_async15/1(real_out1) -> fir_col_async16/1(real1)
  fir_col_async15/2(imag_out1) -> fir_col_async16/2(imag1)
  fir_col_async15/3(real_out2) -> fir_col_async16/3(real2)
  fir_col_async15/4(imag_out2) -> fir_col_async16/4(imag2)
  fir_col_async15/5(real_out3) -> fir_col_async16/5(real3)
  fir_col_async15/6(imag_out3) -> fir_col_async16/6(imag3)
  fir_col_async15/7(real_out4) -> fir_col_async16/7(real4)
  fir_col_async15/8(imag_out4) -> fir_col_async16/8(imag4)
  fir_col_async15/9(real_out5) -> fir_col_async16/9(real5)
  fir_col_async15/10(imag_out5) -> fir_col_async16/10(imag5)
  fir_col_async15/11(real_out6) -> fir_col_async16/11(real6)
  fir_col_async15/12(imag_out6) -> fir_col_async16/12(imag6)
  fir_col_async15/13(real_out7) -> fir_col_async16/13(real7)
  fir_col_async15/14(imag_out7) -> fir_col_async16/14(imag7)
  fir_col_async15/15(real_out8) -> fir_col_async16/15(real8)
  fir_col_async15/16(imag_out8) -> fir_col_async16/16(imag8)
  fir_col_async16/17(real_sum) -> real_sum/17(din16)
  fir_col_async16/18(imag_sum) -> imag_sum/17(din16)
  fir_col_async16/1(real_out1) -> fir_col_async17/1(real1)
  fir_col_async16/2(imag_out1) -> fir_col_async17/2(imag1)
  fir_col_async16/3(real_out2) -> fir_col_async17/3(real2)
  fir_col_async16/4(imag_out2) -> fir_col_async17/4(imag2)
  fir_col_async16/5(real_out3) -> fir_col_async17/5(real3)
  fir_col_async16/6(imag_out3) -> fir_col_async17/6(imag3)
  fir_col_async16/7(real_out4) -> fir_col_async17/7(real4)
  fir_col_async16/8(imag_out4) -> fir_col_async17/8(imag4)
  fir_col_async16/9(real_out5) -> fir_col_async17/9(real5)
  fir_col_async16/10(imag_out5) -> fir_col_async17/10(imag5)
  fir_col_async16/11(real_out6) -> fir_col_async17/11(real6)
  fir_col_async16/12(imag_out6) -> fir_col_async17/12(imag6)
  fir_col_async16/13(real_out7) -> fir_col_async17/13(real7)
  fir_col_async16/14(imag_out7) -> fir_col_async17/14(imag7)
  fir_col_async16/15(real_out8) -> fir_col_async17/15(real8)
  fir_col_async16/16(imag_out8) -> fir_col_async17/16(imag8)
  fir_col_async17/17(real_sum) -> real_sum/18(din17)
  fir_col_async17/18(imag_sum) -> imag_sum/18(din17)
  fir_col_async17/1(real_out1) -> fir_col_async18/1(real1)
  fir_col_async17/2(imag_out1) -> fir_col_async18/2(imag1)
  fir_col_async17/3(real_out2) -> fir_col_async18/3(real2)
  fir_col_async17/4(imag_out2) -> fir_col_async18/4(imag2)
  fir_col_async17/5(real_out3) -> fir_col_async18/5(real3)
  fir_col_async17/6(imag_out3) -> fir_col_async18/6(imag3)
  fir_col_async17/7(real_out4) -> fir_col_async18/7(real4)
  fir_col_async17/8(imag_out4) -> fir_col_async18/8(imag4)
  fir_col_async17/9(real_out5) -> fir_col_async18/9(real5)
  fir_col_async17/10(imag_out5) -> fir_col_async18/10(imag5)
  fir_col_async17/11(real_out6) -> fir_col_async18/11(real6)
  fir_col_async17/12(imag_out6) -> fir_col_async18/12(imag6)
  fir_col_async17/13(real_out7) -> fir_col_async18/13(real7)
  fir_col_async17/14(imag_out7) -> fir_col_async18/14(imag7)
  fir_col_async17/15(real_out8) -> fir_col_async18/15(real8)
  fir_col_async17/16(imag_out8) -> fir_col_async18/16(imag8)
  fir_col_async18/17(real_sum) -> real_sum/19(din18)
  fir_col_async18/18(imag_sum) -> imag_sum/19(din18)
  fir_col_async18/1(real_out1) -> fir_col_async19/1(real1)
  fir_col_async18/2(imag_out1) -> fir_col_async19/2(imag1)
  fir_col_async18/3(real_out2) -> fir_col_async19/3(real2)
  fir_col_async18/4(imag_out2) -> fir_col_async19/4(imag2)
  fir_col_async18/5(real_out3) -> fir_col_async19/5(real3)
  fir_col_async18/6(imag_out3) -> fir_col_async19/6(imag3)
  fir_col_async18/7(real_out4) -> fir_col_async19/7(real4)
  fir_col_async18/8(imag_out4) -> fir_col_async19/8(imag4)
  fir_col_async18/9(real_out5) -> fir_col_async19/9(real5)
  fir_col_async18/10(imag_out5) -> fir_col_async19/10(imag5)
  fir_col_async18/11(real_out6) -> fir_col_async19/11(real6)
  fir_col_async18/12(imag_out6) -> fir_col_async19/12(imag6)
  fir_col_async18/13(real_out7) -> fir_col_async19/13(real7)
  fir_col_async18/14(imag_out7) -> fir_col_async19/14(imag7)
  fir_col_async18/15(real_out8) -> fir_col_async19/15(real8)
  fir_col_async18/16(imag_out8) -> fir_col_async19/16(imag8)
  fir_col_async19/17(real_sum) -> real_sum/20(din19)
  fir_col_async19/18(imag_sum) -> imag_sum/20(din19)
  fir_col_async19/1(real_out1) -> fir_col_async20/1(real1)
  fir_col_async19/2(imag_out1) -> fir_col_async20/2(imag1)
  fir_col_async19/3(real_out2) -> fir_col_async20/3(real2)
  fir_col_async19/4(imag_out2) -> fir_col_async20/4(imag2)
  fir_col_async19/5(real_out3) -> fir_col_async20/5(real3)
  fir_col_async19/6(imag_out3) -> fir_col_async20/6(imag3)
  fir_col_async19/7(real_out4) -> fir_col_async20/7(real4)
  fir_col_async19/8(imag_out4) -> fir_col_async20/8(imag4)
  fir_col_async19/9(real_out5) -> fir_col_async20/9(real5)
  fir_col_async19/10(imag_out5) -> fir_col_async20/10(imag5)
  fir_col_async19/11(real_out6) -> fir_col_async20/11(real6)
  fir_col_async19/12(imag_out6) -> fir_col_async20/12(imag6)
  fir_col_async19/13(real_out7) -> fir_col_async20/13(real7)
  fir_col_async19/14(imag_out7) -> fir_col_async20/14(imag7)
  fir_col_async19/15(real_out8) -> fir_col_async20/15(real8)
  fir_col_async19/16(imag_out8) -> fir_col_async20/16(imag8)
  fir_col_async20/17(real_sum) -> real_sum/21(din20)
  fir_col_async20/18(imag_sum) -> imag_sum/21(din20)
  fir_col_async20/1(real_out1) -> fir_col_async21/1(real1)
  fir_col_async20/2(imag_out1) -> fir_col_async21/2(imag1)
  fir_col_async20/3(real_out2) -> fir_col_async21/3(real2)
  fir_col_async20/4(imag_out2) -> fir_col_async21/4(imag2)
  fir_col_async20/5(real_out3) -> fir_col_async21/5(real3)
  fir_col_async20/6(imag_out3) -> fir_col_async21/6(imag3)
  fir_col_async20/7(real_out4) -> fir_col_async21/7(real4)
  fir_col_async20/8(imag_out4) -> fir_col_async21/8(imag4)
  fir_col_async20/9(real_out5) -> fir_col_async21/9(real5)
  fir_col_async20/10(imag_out5) -> fir_col_async21/10(imag5)
  fir_col_async20/11(real_out6) -> fir_col_async21/11(real6)
  fir_col_async20/12(imag_out6) -> fir_col_async21/12(imag6)
  fir_col_async20/13(real_out7) -> fir_col_async21/13(real7)
  fir_col_async20/14(imag_out7) -> fir_col_async21/14(imag7)
  fir_col_async20/15(real_out8) -> fir_col_async21/15(real8)
  fir_col_async20/16(imag_out8) -> fir_col_async21/16(imag8)
  fir_col_async21/17(real_sum) -> real_sum/22(din21)
  fir_col_async21/18(imag_sum) -> imag_sum/22(din21)
  real_sum/2(dout) -> shift1/1
  imag_sum/2(dout) -> shift2/1
  shift1/1 -> convert1/1
  shift2/1 -> convert2/1
  convert1/1 -> ri_to_c/1
  convert2/1 -> ri_to_c/2
  ri_to_c/1 -> dout/1
  sync_delay/1 -> real_sum/1(sync), imag_sum/1(sync)
  real_sum/1(sync_out) -> sync_out/1
